simulink library "MATH_library"  (R2018b)
settings: Solver=VariableStepAuto  StartTime=0.0  StopTime=10.0  RelTol=1e-3
undefined symbols (not defined in the file): Newton, Raphson
libraries: $bdroot x48, sharedutil x4
(part 2 of 2)

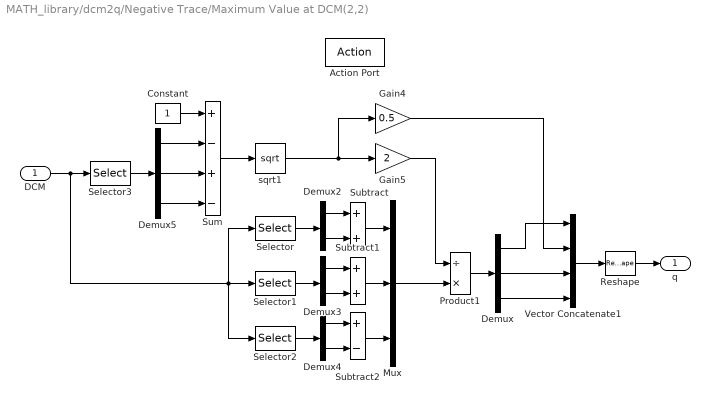
== system MATH_library/dcm2q/Negative Trace/Maximum Value at DCM(2,2) ==
  DCM : Inport
  Action Port : ActionPort  PropagateVarSize=During execution
  Constant : Constant
  Demux : Demux  Outputs=3
  Demux2 : Demux  Outputs=2
  Demux3 : Demux  Outputs=2
  Demux4 : Demux  Outputs=2
  Demux5 : Demux  Outputs=3
  Gain4 : Gain  Gain=0.5  OutDataTypeStr=Inherit: Inherit via back propagation  SaturateOnIntegerOverflow=on  ParamDataTypeStr=Inherit: Same as input
  Gain5 : Gain  Gain=2  OutDataTypeStr=Inherit: Inherit via back propagation  SaturateOnIntegerOverflow=on  ParamDataTypeStr=Inherit: Same as input
  Mux : Mux  Inputs=3
  Product1 : Product  Inputs=/*  SaturateOnIntegerOverflow=on  InputSameDT=on  OutDataTypeStr=Inherit: Same as first input
  Reshape : Reshape  OutputDimensionality=Column vector (2-D)
  Selector : Selector  InputPortWidth=9  IndexOptions=Index vector (dialog)  Indices=[2 4]  OutputSizes=1
  Selector1 : Selector  InputPortWidth=9  IndexOptions=Index vector (dialog)  Indices=[6 8]  OutputSizes=1
  Selector2 : Selector  InputPortWidth=9  IndexOptions=Index vector (dialog)  Indices=[3 7]  OutputSizes=1
  Selector3 : Selector  InputPortWidth=9  IndexOptions=Index vector (dialog)  Indices=[1 5 9]  OutputSizes=1
  Subtract : Sum
  Subtract1 : Sum
  Subtract2 : Sum  Inputs=+-
  Sum : Sum  Inputs=+-+-  SaturateOnIntegerOverflow=on  InputSameDT=on  OutDataTypeStr=Inherit: Same as first input
  Vector Concatenate1 : Concatenate  NumInputs=4
  sqrt1 : Sqrt  AlgorithmType=Newton-Raphson  SaturateOnIntegerOverflow=on
  q : Outport
  wires:
  Reshape/1 -> q/1
  Vector Concatenate1/1 -> Reshape/1
  Demux2/1 -> Subtract/1
  Demux2/2 -> Subtract/2
  Subtract2/1 -> Mux/3
  Demux5/2 -> Sum/3
  Selector3/1 -> Demux5/1
  Subtract1/1 -> Mux/2
  Selector/1 -> Demux2/1
  DCM/1 -> Selector/1, Selector2/1, Selector1/1, Selector3/1
  Demux3/1 -> Subtract1/1
  Subtract/1 -> Mux/1
  Demux3/2 -> Subtract1/2
  Demux4/1 -> Subtract2/1
  Demux5/1 -> Sum/2
  sqrt1/1 -> Gain4/1, Gain5/1
  Sum/1 -> sqrt1/1
  Mux/1 -> Product1/2
  Selector1/1 -> Demux3/1
  Gain5/1 -> Product1/1
  Selector2/1 -> Demux4/1
  Demux5/3 -> Sum/4
  Demux4/2 -> Subtract2/2
  Constant/1 -> Sum/1
  Product1/1 -> Demux/1
  Demux/3 -> Vector Concatenate1/4
  Demux/2 -> Vector Concatenate1/3
  Demux/1 -> Vector Concatenate1/1
  Gain4/1 -> Vector Concatenate1/2

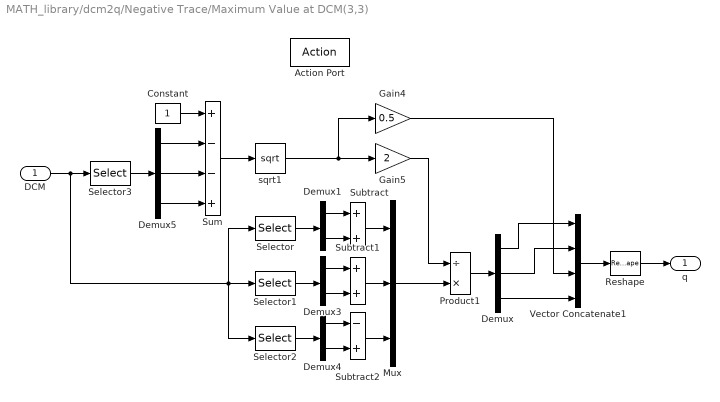
== system MATH_library/dcm2q/Negative Trace/Maximum Value at DCM(3,3) ==
  DCM : Inport
  Action Port : ActionPort  PropagateVarSize=During execution
  Constant : Constant
  Demux : Demux  Outputs=3
  Demux1 : Demux  Outputs=2
  Demux3 : Demux  Outputs=2
  Demux4 : Demux  Outputs=2
  Demux5 : Demux  Outputs=3
  Gain4 : Gain  Gain=0.5  OutDataTypeStr=Inherit: Inherit via back propagation  SaturateOnIntegerOverflow=on  ParamDataTypeStr=Inherit: Same as input
  Gain5 : Gain  Gain=2  OutDataTypeStr=Inherit: Inherit via back propagation  SaturateOnIntegerOverflow=on  ParamDataTypeStr=Inherit: Same as input
  Mux : Mux  Inputs=3
  Product1 : Product  Inputs=/*  SaturateOnIntegerOverflow=on  InputSameDT=on  OutDataTypeStr=Inherit: Same as first input
  Reshape : Reshape  OutputDimensionality=Column vector (2-D)
  Selector : Selector  InputPortWidth=9  IndexOptions=Index vector (dialog)  Indices=[3 7]  OutputSizes=1
  Selector1 : Selector  InputPortWidth=9  IndexOptions=Index vector (dialog)  Indices=[6 8]  OutputSizes=1
  Selector2 : Selector  InputPortWidth=9  IndexOptions=Index vector (dialog)  Indices=[2 4]  OutputSizes=1
  Selector3 : Selector  InputPortWidth=9  IndexOptions=Index vector (dialog)  Indices=[1 5 9]  OutputSizes=1
  Subtract : Sum
  Subtract1 : Sum
  Subtract2 : Sum  Inputs=-+
  Sum : Sum  Inputs=+--+  SaturateOnIntegerOverflow=on  InputSameDT=on  OutDataTypeStr=Inherit: Same as first input
  Vector Concatenate1 : Concatenate  NumInputs=4
  sqrt1 : Sqrt  AlgorithmType=Newton-Raphson  SaturateOnIntegerOverflow=on
  q : Outport
  wires:
  Reshape/1 -> q/1
  Selector/1 -> Demux1/1
  Subtract2/1 -> Mux/3
  Gain5/1 -> Product1/1
  Demux5/2 -> Sum/3
  Selector1/1 -> Demux3/1
  Subtract/1 -> Mux/1
  Demux3/1 -> Subtract1/1
  Mux/1 -> Product1/2
  Demux4/2 -> Subtract2/2
  Sum/1 -> sqrt1/1
  Subtract1/1 -> Mux/2
  Vector Concatenate1/1 -> Reshape/1
  Demux/3 -> Vector Concatenate1/4
  Demux5/3 -> Sum/4
  Demux4/1 -> Subtract2/1
  Demux3/2 -> Subtract1/2
  Demux5/1 -> Sum/2
  Constant/1 -> Sum/1
  Demux/1 -> Vector Concatenate1/1
  sqrt1/1 -> Gain4/1, Gain5/1
  DCM/1 -> Selector/1, Selector2/1, Selector1/1, Selector3/1
  Demux1/2 -> Subtract/2
  Product1/1 -> Demux/1
  Demux1/1 -> Subtract/1
  Selector2/1 -> Demux4/1
  Selector3/1 -> Demux5/1
  Gain4/1 -> Vector Concatenate1/3
  Demux/2 -> Vector Concatenate1/2
